simulink model "test"  (R2013b)
settings: Solver=ode45  StartTime=0.0  StopTime=10.0  RelTol=1e-3
libraries: xbsIndex_r4 x28, xps_library x1
settings Model: Creator=root  LastModifiedBy=root

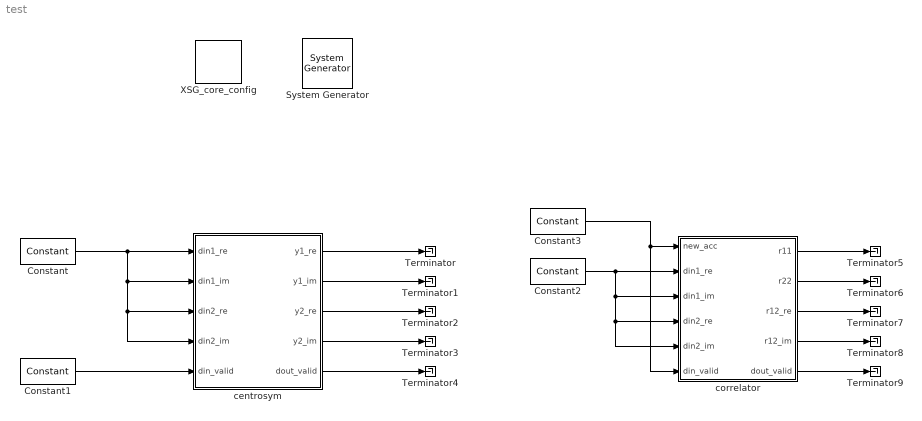
== system test ==
  " System Generator" : xbsIndex_r4/ System Generator  Tag=genX  xilinxfamily=Kintex7  part=xc7k325t  speed=-3  package=fbg676  synthesis_tool=XST  clock_wrapper=Clock Enables  directory=./netlist  proj_type=Project Navigator  Synth_file=XST Defaults  Impl_file=ISE Defaults  testbench=off  simulink_period=1  sysclk_period=10  dcm_input_clock_period=10  incr_netlist=off  trim_vbits=Everywhere in SubSystem  dbl_ovrd=According to Block Masks  core_generation=According to Block Masks  run_coregen=off  deprecated_control=off  eval_field=0  block_type=sysgen
  Constant : xbsIndex_r4/Constant  const=1  gui_display_data_type=Fixed-point  arith_type=Signed (2's comp)  n_bits=18  bin_pt=14  preci_type=Single  exp_width=8  frac_width=24  explicit_period=on  period=1  equ=P=C  opselect=C  inp2=PCIN>>17  opr=+  inp1=P  carry=CIN  dbl_ovrd=off  block_type=constant
  Constant1 : xbsIndex_r4/Constant  const=1  gui_display_data_type=Boolean  arith_type=Boolean  n_bits=18  bin_pt=14  preci_type=Single  exp_width=8  frac_width=24  explicit_period=on  period=1  equ=P=C  opselect=C  inp2=PCIN>>17  opr=+  inp1=P  carry=CIN  dbl_ovrd=off  block_type=constant
  Constant2 : xbsIndex_r4/Constant  const=1  gui_display_data_type=Fixed-point  arith_type=Signed (2's comp)  n_bits=18  bin_pt=14  preci_type=Single  exp_width=8  frac_width=24  explicit_period=on  period=1  equ=P=C  opselect=C  inp2=PCIN>>17  opr=+  inp1=P  carry=CIN  dbl_ovrd=off  block_type=constant
  Constant3 : xbsIndex_r4/Constant  const=1  gui_display_data_type=Boolean  arith_type=Boolean  n_bits=18  bin_pt=14  preci_type=Single  exp_width=8  frac_width=24  explicit_period=on  period=1  equ=P=C  opselect=C  inp2=PCIN>>17  opr=+  inp1=P  carry=CIN  dbl_ovrd=off  block_type=constant
  Terminator{,1..9} (10 alike) : Terminator
  XSG_core_config : xps_library/XSG_core_config  Tag=xps:xsg  hw_sys=ROACH2:sx475t  clk_src=sys_clk  ROACH_clk_src=sys_clk  ROACH2_clk_src=sys_clk  MKDIG_clk_src=sys_clk  clk_rate=100  sample_period=1  synthesis_tool=XST
  centrosym : Subsystem  mask{din_width=18, din_point=17}
      mask prompts: din_width "din width"; din_point "din point"
  correlator : Subsystem  mask{din_width=19, din_point=17, vector_len=512, acc_width=20, acc_point=16, dout_width=32}
      mask prompts: din_width "din width"; din_point "din point"; vector_len "vector len"; acc_width "accumulator width"; acc_point "accumulator point"; dout_width "dout width"
  wires:
  Constant/1 -> centrosym/2(din1_im), centrosym/3(din2_re), centrosym/4(din2_im), centrosym/1(din1_re)
  Constant1/1 -> centrosym/5(din_valid)
  centrosym/1(y1_re) -> Terminator/1
  centrosym/2(y1_im) -> Terminator1/1
  centrosym/3(y2_re) -> Terminator2/1
  centrosym/4(y2_im) -> Terminator3/1
  centrosym/5(dout_valid) -> Terminator4/1
  Constant2/1 -> correlator/3(din1_im), correlator/5(din2_im), correlator/4(din2_re), correlator/2(din1_re)
  Constant3/1 -> correlator/6(din_valid), correlator/1(new_acc)
  correlator/1(r11) -> Terminator5/1
  correlator/2(r22) -> Terminator6/1
  correlator/3(r12_re) -> Terminator7/1
  correlator/4(r12_im) -> Terminator8/1
  correlator/5(dout_valid) -> Terminator9/1

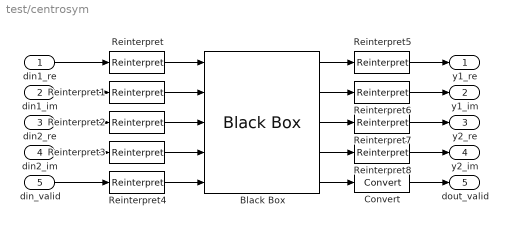
== system test/centrosym ==
  din1_re : Inport
  din1_im : Inport  Port=2
  din2_re : Inport  Port=3
  din2_im : Inport  Port=4
  din_valid : Inport  Port=5
  Black Box : xbsIndex_r4/Black Box  init_code=centrosym_matrix_config  sim_method=Inactive  verbose=off  block_type=blackbox2
  Convert : xbsIndex_r4/Convert  gui_display_data_type=Boolean  arith_type=Boolean  n_bits=3  bin_pt=0  float_type=Single  exp_bits=8  fraction_bits=24  quantization=Truncate  overflow=Wrap  en=off  latency=0  dbl_ovrd=off  pipeline=off  block_type=convert
      settings: block_version=11.4
  Reinterpret{,1..4} (5 alike) : xbsIndex_r4/Reinterpret  force_arith_type=on  arith_type=Unsigned  force_bin_pt=on  bin_pt=0  block_type=reinterpret
  Reinterpret{5..8} (4 alike) : xbsIndex_r4/Reinterpret  force_arith_type=on  arith_type="Signed  (2's comp)"  force_bin_pt=on  bin_pt=din_point  block_type=reinterpret
  y1_re : Outport
  y1_im : Outport  Port=2
  y2_re : Outport  Port=3
  y2_im : Outport  Port=4
  dout_valid : Outport  Port=5
  wires:
  din1_re/1 -> Reinterpret/1
  din2_re/1 -> Reinterpret2/1
  din2_im/1 -> Reinterpret3/1
  Black Box/3 -> Reinterpret7/1
  Black Box/1 -> Reinterpret5/1
  Black Box/2 -> Reinterpret6/1
  din1_im/1 -> Reinterpret1/1
  Black Box/4 -> Reinterpret8/1
  din_valid/1 -> Reinterpret4/1
  Black Box/5 -> Convert/1
  Reinterpret/1 -> Black Box/1
  Reinterpret1/1 -> Black Box/2
  Reinterpret3/1 -> Black Box/4
  Reinterpret2/1 -> Black Box/3
  Reinterpret4/1 -> Black Box/5
  Reinterpret5/1 -> y1_re/1
  Reinterpret6/1 -> y1_im/1
  Reinterpret7/1 -> y2_re/1
  Reinterpret8/1 -> y2_im/1
  Convert/1 -> dout_valid/1

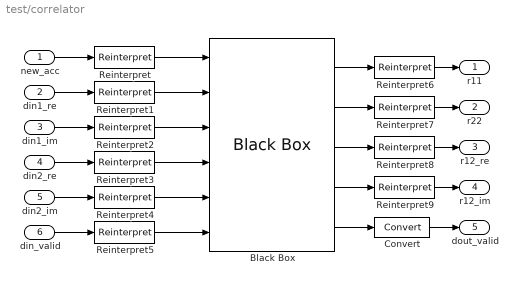
== system test/correlator ==
  new_acc : Inport
  din1_re : Inport  Port=2
  din1_im : Inport  Port=3
  din2_re : Inport  Port=4
  din2_im : Inport  Port=5
  din_valid : Inport  Port=6
  Black Box : xbsIndex_r4/Black Box  init_code=correlator_config  sim_method=Inactive  verbose=off  block_type=blackbox2
  Convert : xbsIndex_r4/Convert  gui_display_data_type=Boolean  arith_type=Boolean  n_bits=3  bin_pt=0  float_type=Single  exp_bits=8  fraction_bits=24  quantization=Truncate  overflow=Wrap  en=off  latency=0  dbl_ovrd=off  pipeline=off  block_type=convert
      settings: block_version=11.4
  Reinterpret{,1..5} (6 alike) : xbsIndex_r4/Reinterpret  force_arith_type=on  arith_type=Unsigned  force_bin_pt=on  bin_pt=0  block_type=reinterpret
  Reinterpret6 : xbsIndex_r4/Reinterpret  force_arith_type=on  arith_type=Unsigned  force_bin_pt=on  bin_pt=acc_point  block_type=reinterpret
  Reinterpret7 : xbsIndex_r4/Reinterpret  force_arith_type=on  arith_type=Unsigned  force_bin_pt=on  bin_pt=acc_point  block_type=reinterpret
  Reinterpret8 : xbsIndex_r4/Reinterpret  force_arith_type=on  arith_type="Signed  (2's comp)"  force_bin_pt=on  bin_pt=acc_point  block_type=reinterpret
  Reinterpret9 : xbsIndex_r4/Reinterpret  force_arith_type=on  arith_type="Signed  (2's comp)"  force_bin_pt=on  bin_pt=acc_point  block_type=reinterpret
  r11 : Outport
  r22 : Outport  Port=2
  r12_re : Outport  Port=3
  r12_im : Outport  Port=4
  dout_valid : Outport  Port=5
  wires:
  new_acc/1 -> Reinterpret/1
  din1_re/1 -> Reinterpret1/1
  din2_re/1 -> Reinterpret3/1
  din1_im/1 -> Reinterpret2/1
  din2_im/1 -> Reinterpret4/1
  Black Box/4 -> Reinterpret9/1
  Black Box/3 -> Reinterpret8/1
  din_valid/1 -> Reinterpret5/1
  Black Box/1 -> Reinterpret6/1
  Black Box/2 -> Reinterpret7/1
  Black Box/5 -> Convert/1
  Reinterpret/1 -> Black Box/1
  Reinterpret1/1 -> Black Box/2
  Reinterpret2/1 -> Black Box/3
  Reinterpret3/1 -> Black Box/4
  Reinterpret4/1 -> Black Box/5
  Reinterpret5/1 -> Black Box/6
  Reinterpret6/1 -> r11/1
  Reinterpret7/1 -> r22/1
  Reinterpret8/1 -> r12_re/1
  Reinterpret9/1 -> r12_im/1
  Convert/1 -> dout_valid/1
